simulink model "Exo_Body_Model"  (R2021a)
settings: Solver=FixedStepAuto  StartTime=0.0  StopTime=10  FixedStep=0.001  RelTol=1e-3  AbsTol=1e-3  EnableMultiTasking=on
values from neighbouring files (symbols this model uses):
  g = 9.81    [Preimplementation.m]
  kd = -20    [Preimplementation.m]
  ki = -50    [Preimplementation.m]
  kp = -50    [Preimplementation.m]
  ShoulderAdduction = deg2rad(-45)    [Preimplementation.m]
  ShoulderExtension = deg2rad(45)    [Preimplementation.m]
  thetaEE_Ref = deg2rad(90)    [Preimplementation.m]
  Wl = 30    [Preimplementation.m]
undefined symbols (not defined in the file or in its folder): X, Y, Z
libraries: sm_lib x29, nesl_utility x7
(part 1 of 2)
settings Model: Creator=Shivam Jaiswal  LastModifiedBy=Shivam Jaiswal
settings SolverCC: AutoScaleAbsTol=off
settings DataIOCC: LimitDataPoints=on  MaxDataPoints=10000
settings OptimizationCC: LifeSpan=inf
settings DebuggingCC: AllowSymbolicDim=off  SFUnexpectedBacktrackingDiag=warning  SFNoUnconditionalDefaultTransitionDiag=warning  SFExecutionAtInitializationDiag=none  SFMachineParentedDataDiag=warning  ArithmeticOperatorsInVariantConditions=warning
settings SFSimCC: SimUseLocalCustomCode=off  CustomCodeUndefinedFunction=UseInterfaceOnly
settings RTWCC: RTWUseLocalCustomCode=off
settings CodeAppCC: StateflowObjectComments=on
settings GRTTargetCC: TargetLangStandard=C89/C90 (ANSI)
settings ConfigComp: CovMetricSettings=dw  CovSaveCumulativeToWorkspaceVar=on  CovSaveSingleToWorkspaceVar=on  CovExternalEMLEnable=off  CovSFcnEnable=off
settings SimscapeCC: SimscapeLogType=all  SimscapeLogSimulationStatistics=on  SimscapeLogDataHistory=10000

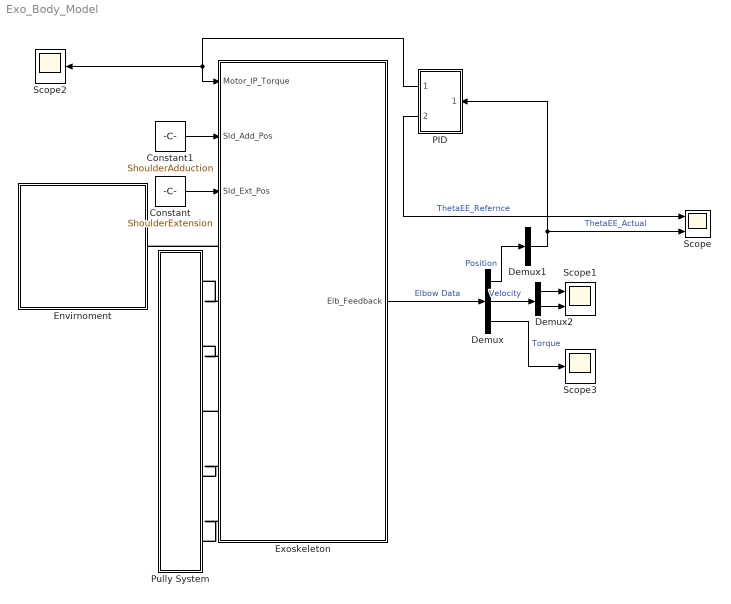
== system Exo_Body_Model ==
  Constant : Constant  Value=ShoulderExtension
  Constant1 : Constant  Value=ShoulderAdduction
  Demux : Demux  Outputs=3
  Demux1 : Demux  Outputs=1
  Demux2 : Demux  Outputs=2
  Envirnoment : Subsystem
  Exoskeleton : Subsystem
  PID : Subsystem
  Pully System : Subsystem
  Scope : Scope  NumInputPorts=2
  Scope1 : Scope  NumInputPorts=2
  Scope2 : Scope
  Scope3 : Scope
  wires:
  Constant/1 -> Exoskeleton/3(Sld_Ext_Pos)
  Constant1/1 -> Exoskeleton/2(Sld_Add_Pos)
  Exoskeleton/1(Elb_Feedback) -> Demux/1  "Elbow Data"
  Demux/2 -> Demux2/1  "Velocity"
  Demux/1 -> Demux1/1  "Position"
  Demux2/1 -> Scope1/1
  Demux2/2 -> Scope1/2
  Demux1/1 -> PID/1(1), Scope/2  "ThetaEE_Actual"
  Demux/3 -> Scope3/1  "Torque"
  PID/1(Out1) -> Exoskeleton/1(Motor_IP_Torque), Scope2/1
  PID/2(Out2) -> Scope/1  "ThetaEE_Refernce"
  connections:
  Exoskeleton/LConn2 -- Pully System/LConn1
  Exoskeleton/LConn3 -- Pully System/LConn2
  Exoskeleton/LConn4 -- Pully System/LConn3
  Exoskeleton/LConn5 -- Pully System/LConn4
  Exoskeleton/LConn6 -- Pully System/LConn5
  Exoskeleton/LConn1 -- Envirnoment/RConn1

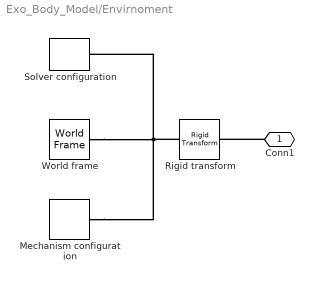
== system Exo_Body_Model/Envirnoment ==
  Mechanism configuration : sm_lib/Utilities/Mechanism Configuration  UniformGravity=Constant  GravityVector=[0 0 -g]  GravityVectorUnits=m/s^2  GravityUnits=m/s^2  LinearizationDelta=0.001  JointModeTransitionNonlinearIterations=2
  Rigid transform : sm_lib/Frames and Transforms/Rigid Transform  TranslationMethod=None  TranslationStandardOffset=0  TranslationLengthUnit=m  TranslationStandardAxis=+Z  TranslationCartesianOffset=[0 0 0]  TranslationROffset=0  TranslationROffsetUnits=m  TranslationZOffset=0  TranslationZOffsetUnits=m  TranslationThetaOffset=0  TranslationThetaOffsetUnits=deg  RotationMethod=StandardAxis  RotationAngleUnits=deg  RotationStandardAxis=+X  RotationAngle=0  RotationArbitraryAxis=[0 0 1]  FollAlignAxisA=+X  BaseAlignAxisA=+Y  FollAlignAxisB=+Y  BaseAlignAxisB=+Z  RotationSequenceAxes=FollowerAxes  RotationSequence=XYX  RotationSequenceAngles=[0 0 0]  RotationSequenceAnglesUnits=deg  RotationMatrix=[1 0 0; 0 1 0; 0 0 1]
  Solver configuration : nesl_utility/Solver Configuration  PhysicalDomain=network_engine_domain  SubClassName=solver  LeftPortType=input  RightPortType=generic  Tones=[]  Harmonics=[]  SimulateNoise=off  Profile=off  UseLocalSampling=off  EnableSwitchedLinearOptims=on  FrequencyDomain=off  UseCCode=off  RelTol=0.001  AbsTol=1e-06  MinStep=1e-09  ToWorkspace=off  RevertToSquareIcSolve=off  NumHomotopyIterations=100  PhasorMode=off  PhasorModeNumHarmonics=1  DoDC=off  ResidualTolerance=1e-09  UseLocalSolver=off  LocalSolverChoice=NE_BACKWARD_EULER_ADVANCER  LocalSolverSampleTime=0.001  DoFixedCost=off  MaxNonlinIter=3  MaxModeIter=2  ComputeImpulses=off  ImpulseIterations=2  LinearAlgebra=Sparse  EquationFormulation=NE_TIME_EF  DelaysMemoryBudget=1024  AutomaticFiltering=on  FilteringTimeConstant=0.001  PartitionStorageMethod=AS_NEEDED  PartitionMemoryBudget=1024  PartitionMethod=FAST
      settings: SourceProductBaseCode=PW,SS
  World frame : sm_lib/Frames and Transforms/World Frame
  Conn1 : PMIOPort  Side=Right
  connections:
  World frame/RConn1 -- Solver configuration/RConn1 -- Rigid transform/LConn1 -- Mechanism configuration/RConn1
  Conn1/RConn1 -- Rigid transform/RConn1
